simulink model "system_layout"  (R2024b)
settings: Solver=VariableStepAuto  StartTime=0.0  StopTime=10.0  RelTol=1e-3
settings Model: Creator=The MathWorks, Inc.  LastModifiedBy=hp
settings SolverCC: AlgebraicLoopSolver=TrustRegion
settings DataIOCC: ReturnWorkspaceOutputs=off
settings DebuggingCC: BusObjectLabelMismatch=none  RootOutportRequireBusObject=none  PregeneratedLibrarySubsystemCodeDiagnostic=none  ArithmeticOperatorsInVariantConditions=warning
settings ModelReferenceCC: EnableRefExpFcnMdlSchedulingChecks=on
settings SFSimCC: SimUseLocalCustomCode=off
settings RTWCC: RTWUseLocalCustomCode=off  GPUComputeCapability=3.5

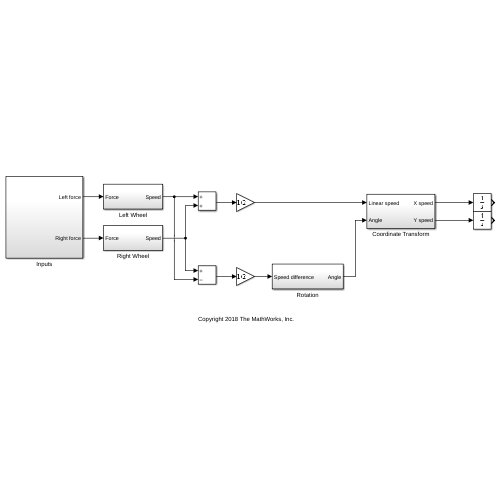
[thumbnail: Simulink's stored preview of the top-level diagram]
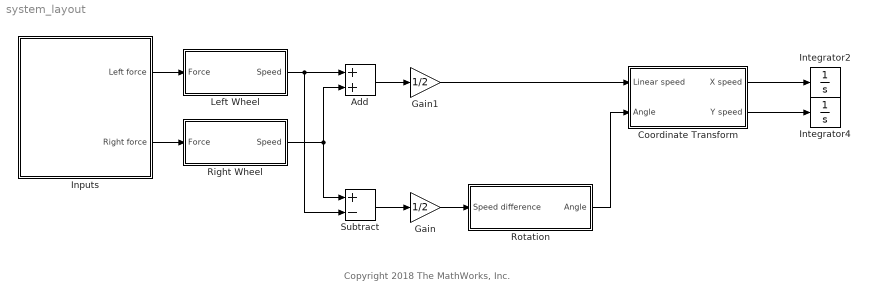
== system system_layout ==
  note: Copyright 2018 The MathWorks, Inc.
  Add : Sum
  Coordinate Transform : Subsystem
  Gain : Gain  Gain=1/2
  Gain1 : Gain  Gain=1/2
  Inputs : Subsystem
  Integrator2 : Integrator
  Integrator4 : Integrator
  Left Wheel : Subsystem
  Right Wheel : Subsystem
  Rotation : Subsystem
  Subtract : Sum  Inputs=+-
  wires:
  Inputs/1(Left force) -> Left Wheel/1(Force)
  Inputs/2(Right force) -> Right Wheel/1(Force)
  Coordinate Transform/1(X speed) -> Integrator2/1
  Coordinate Transform/2(Y speed) -> Integrator4/1
  Left Wheel/1(Speed) -> Subtract/2, Add/1
  Right Wheel/1(Speed) -> Subtract/1, Add/2
  Rotation/1(Angle) -> Coordinate Transform/2(Angle)
  Subtract/1 -> Gain/1
  Gain/1 -> Rotation/1(Speed difference)
  Add/1 -> Gain1/1
  Gain1/1 -> Coordinate Transform/1(Linear speed)

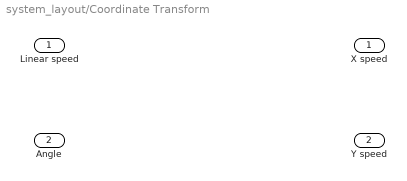
== system system_layout/Coordinate Transform ==
  Linear speed : Inport
  Angle : Inport  Port=2
  X speed : Outport  VectorParamsAs1DForOutWhenUnconnected=off
  Y speed : Outport  Port=2  VectorParamsAs1DForOutWhenUnconnected=off

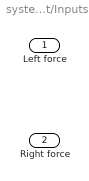
== system system_layout/Inputs ==
  Left force : Outport  VectorParamsAs1DForOutWhenUnconnected=off
  Right force : Outport  Port=2  VectorParamsAs1DForOutWhenUnconnected=off

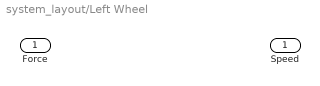
== system system_layout/Left Wheel ==
  Force : Inport
  Speed : Outport  VectorParamsAs1DForOutWhenUnconnected=off

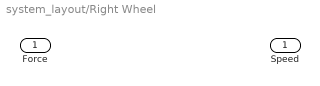
== system system_layout/Right Wheel ==
  Force : Inport
  Speed : Outport  VectorParamsAs1DForOutWhenUnconnected=off

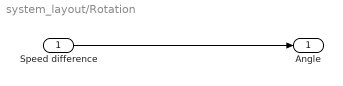
== system system_layout/Rotation ==
  Speed difference : Inport
  Angle : Outport  VectorParamsAs1DForOutWhenUnconnected=off
  wires:
  Speed difference/1 -> Angle/1
